simulink model "Q13dist"  (R2018a)
settings: Solver=VariableStepAuto  StartTime=0.0  StopTime=100  RelTol=1e-3
values from neighbouring files (symbols this model uses):
  A = [0.110571547291 0.471247754055 0.0249955131485 2.58943408161e-06 -0.326108592505 0.861622655316 0.0987425683373 1.02293307698e-05 -0.0747829687831 -0.0317325850518 0.998316867847 0.000207017546418 ... (16 elements, 4x4)]    [Q6.mat]    (also in SteelMillControl10.m = DiscPlant.A; SteelMillControl11.m = DiscPlant.A; SteelMillControl12.m = DiscPlant.A; SteelMillControl12lqr.m = DiscPlant.A)
  B = [0.00184081153928 0.000781109785891 4.14309453057e-05 4.29207838905e-09]    [Q6.mat]    (also in SteelMillControl10.m = DiscPlant.B; SteelMillControl11.m = DiscPlant.B; SteelMillControl12.m = DiscPlant.B; SteelMillControl12lqr.m = DiscPlant.B)
  C = [6.47358520402e-07 2.55733269246e-06 5.17543866044e-05 0.5]    [Q6.mat]    (also in SteelMillControl10.m = DiscPlant.C; SteelMillControl11.m = DiscPlant.C; SteelMillControl12.m = DiscPlant.C; SteelMillControl12lqr.m = DiscPlant.C)
  h = 9    [OlaSoup.m]    (also in Q3.mat = 0.0153022172533; Q6.mat = 0.03257469729; Q9disc.mat = 0.532796640949; SteelMillControl11.m = stepRes.RiseTime/11)
  xinit = [-17 5 -8 0.5]    [Q6.mat]    (also in SteelMillControl10.m = [0 0 0 0]; SteelMillControl11.m = [0 0 0 0]; SteelMillControl12.m = [0 0 0 0]; SteelMillControl12lqr.m = [0 0 0 0])
undefined symbols (not defined in the file or in its folder): Ac, Bc, Cc, Dc
settings Model: Creator=bakos  LastModifiedBy=bakos
settings SolverCC: DecoupledContinuousIntegration=on  MinimalZcImpactIntegration=on

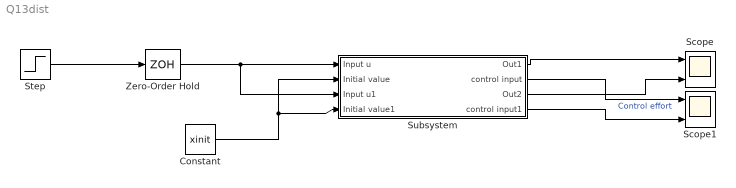
== system Q13dist ==
  Constant : Constant  Value=xinit
  Scope : Scope  NumInputPorts=2
  Scope1 : Scope  NumInputPorts=2
  Step : Step  Time=0  SampleTime=0
  Subsystem : Subsystem
  Zero-Order Hold : ZeroOrderHold  SampleTime=h
  wires:
  Subsystem/1(Out1) -> Scope/1
  Constant/1 -> Subsystem/4(Initial value1), Subsystem/2(Initial value)
  Zero-Order Hold/1 -> Subsystem/3(Input u1), Subsystem/1(Input u)
  Step/1 -> Zero-Order Hold/1
  Subsystem/2(control input) -> Scope1/1  "Control effort"
  Subsystem/4(control input1) -> Scope1/2
  Subsystem/3(Out2) -> Scope/2

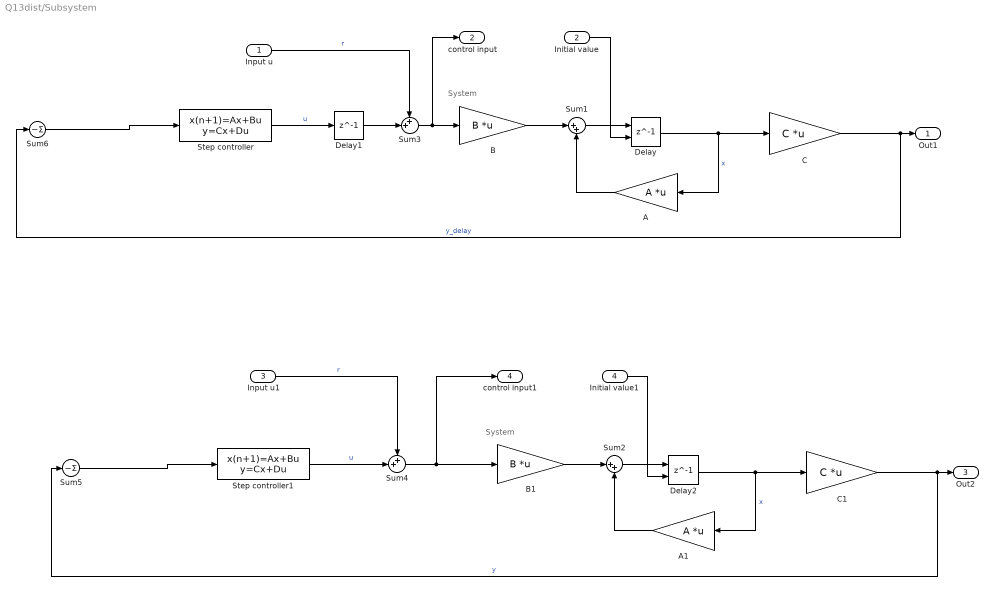
== system Q13dist/Subsystem ==
  note: System
  note: System
  Input u : Inport
  Initial value : Inport  Port=2
  Input u1 : Inport  Port=3
  Initial value1 : Inport  Port=4
  A : Gain  Gain=A  Multiplication=Matrix(K*u)
  A1 : Gain  Gain=A  Multiplication=Matrix(K*u)
  B : Gain  Gain=B  Multiplication=Matrix(K*u)
  B1 : Gain  Gain=B  Multiplication=Matrix(K*u)
  C : Gain  Gain=C  Multiplication=Matrix(K*u)
  C1 : Gain  Gain=C  Multiplication=Matrix(K*u)
  Delay : Delay  DelayLength=1  InitialConditionSource=Input port  InitialCondition=0  SampleTime=h
      settings: InputPortMap=u0,p4
  Delay1 : Delay  DelayLength=1  InitialCondition=0
  Delay2 : Delay  DelayLength=1  InitialConditionSource=Input port  InitialCondition=0  SampleTime=h
      settings: InputPortMap=u0,p4
  Step controller : DiscreteStateSpace  A=Ac  B=Bc  C=Cc  D=Dc  SampleTime=h
  Step controller1 : DiscreteStateSpace  A=Ac  B=Bc  C=Cc  D=Dc  SampleTime=h
  Sum1 : Sum  Inputs=|++
  Sum2 : Sum  Inputs=|++
  Sum3 : Sum  Inputs=++|
  Sum4 : Sum  Inputs=++|
  Sum5 : Sum  Inputs=|-|
  Sum6 : Sum  Inputs=|-|
  Out1 : Outport
  control input : Outport  Port=2
  Out2 : Outport  Port=3
  control input1 : Outport  Port=4
  wires:
  B/1 -> Sum1/1
  Sum1/1 -> Delay/1
  Delay/1 -> A/1, C/1  "x"
  A/1 -> Sum1/2
  Initial value/1 -> Delay/2
  C/1 -> Sum6/1, Out1/1  "y_delay"
  C1/1 -> Sum5/1, Out2/1  "y"
  A1/1 -> Sum2/2
  Delay2/1 -> A1/1, C1/1  "x"
  Sum2/1 -> Delay2/1
  B1/1 -> Sum2/1
  Initial value1/1 -> Delay2/2
  Step controller/1 -> Delay1/1  "u"
  Input u1/1 -> Sum4/1  "r"
  Sum5/1 -> Step controller1/1
  Input u/1 -> Sum3/1  "r"
  Sum6/1 -> Step controller/1
  Delay1/1 -> Sum3/2
  Sum3/1 -> B/1, control input/1
  Step controller1/1 -> Sum4/2  "u"
  Sum4/1 -> control input1/1, B1/1
